simulink model "pid_teta_x"  (R2017b)
settings: Solver=VariableStepAuto  StartTime=0.0  StopTime=3  RelTol=1e-3
libraries: simulink_extras x4, simulink x2
settings Model: Creator=Iman  LastModifiedBy=Iman

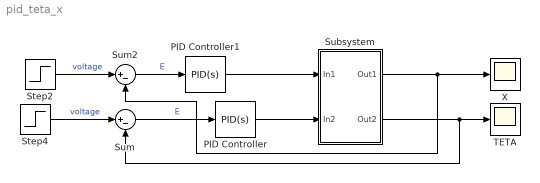
== system pid_teta_x ==
  PID Controller : simulink/Continuous/PID Controller  Controller=PID  TimeDomain=Continuous-time  SampleTime=-1  IntegratorMethod=Forward Euler  FilterMethod=Forward Euler  Form=Parallel  UseFilter=on  ControllerParametersSource=internal  P=-5528615749.16479  I=-14443726305.4223  D=1766735.00522136  N=3129.2840934411  InitialConditionSource=internal  InitialConditionForIntegrator=0  InitialConditionForFilter=0  ExternalReset=none  LimitOutput=off  UpperSaturationLimit=inf  LowerSaturationLimit=-inf  LinearizeAsGain=on  AntiWindupMode=none  Kb=1  TrackingMode=off  Kt=1  PParamMin=[]  PParamMax=[]  IParamMin=[]  IParamMax=[]  DParamMin=[]  DParamMax=[]  NParamMin=[]  NParamMax=[]  KbParamMin=[]  KbParamMax=[]  KtParamMin=[]  KtParamMax=[]  POutMin=[]  POutMax=[]  IOutMin=[]  IOutMax=[]  DOutMin=[]  DOutMax=[]  NOutMin=[]  NOutMax=[]  KbOutMin=[]  KbOutMax=[]  KtOutMin=[]  KtOutMax=[]  IntegratorOutMin=[]  IntegratorOutMax=[]  FilterOutMin=[]  FilterOutMax=[]  SumOutMin=[]  SumOutMax=[]  SumI1OutMin=[]  SumI1OutMax=[]  SumI2OutMin=[]  SumI2OutMax=[]  SumI3OutMin=[]  SumI3OutMax=[]  SumDOutMin=[]  SumDOutMax=[]  SaturationOutMin=[]  SaturationOutMax=[]  IntegratorContinuousStateAttributes=''  IntegratorStateMustResolveToSignalObject=off  IntegratorRTWStateStorageClass=Auto  FilterContinuousStateAttributes=''  FilterStateMustResolveToSignalObject=off  FilterRTWStateStorageClass=Auto  DifferentiatorICPrevScaledInput=0  DifferentiatorOutMin=[]  DifferentiatorOutMax=[]  InitialConditionSetting=State (most efficient)  FilterDiffOutCoefMin=[]  FilterDiffOutCoefMax=[]  SumDenOutMin=[]  SumDenOutMax=[]  SumNumOutMin=[]  SumNumOutMax=[]  ReciprocalOutMin=[]  ReciprocalOutMax=[]  DivideOutMin=[]  DivideOutMax=[]  TunerSelectOption=Transfer Function Based (PID Tuner App)
  PID Controller1 : simulink/Continuous/PID Controller  Controller=PID  TimeDomain=Continuous-time  SampleTime=-1  IntegratorMethod=Forward Euler  FilterMethod=Forward Euler  Form=Parallel  UseFilter=on  ControllerParametersSource=internal  P=85.1454280076779  I=92.389206029507  D=18.0340374207708  N=3627.1106134896  InitialConditionSource=internal  InitialConditionForIntegrator=0  InitialConditionForFilter=0  ExternalReset=none  LimitOutput=off  UpperSaturationLimit=inf  LowerSaturationLimit=-inf  LinearizeAsGain=on  AntiWindupMode=none  Kb=1  TrackingMode=off  Kt=1  PParamMin=[]  PParamMax=[]  IParamMin=[]  IParamMax=[]  DParamMin=[]  DParamMax=[]  NParamMin=[]  NParamMax=[]  KbParamMin=[]  KbParamMax=[]  KtParamMin=[]  KtParamMax=[]  POutMin=[]  POutMax=[]  IOutMin=[]  IOutMax=[]  DOutMin=[]  DOutMax=[]  NOutMin=[]  NOutMax=[]  KbOutMin=[]  KbOutMax=[]  KtOutMin=[]  KtOutMax=[]  IntegratorOutMin=[]  IntegratorOutMax=[]  FilterOutMin=[]  FilterOutMax=[]  SumOutMin=[]  SumOutMax=[]  SumI1OutMin=[]  SumI1OutMax=[]  SumI2OutMin=[]  SumI2OutMax=[]  SumI3OutMin=[]  SumI3OutMax=[]  SumDOutMin=[]  SumDOutMax=[]  SaturationOutMin=[]  SaturationOutMax=[]  IntegratorContinuousStateAttributes=''  IntegratorStateMustResolveToSignalObject=off  IntegratorRTWStateStorageClass=Auto  FilterContinuousStateAttributes=''  FilterStateMustResolveToSignalObject=off  FilterRTWStateStorageClass=Auto  DifferentiatorICPrevScaledInput=0  DifferentiatorOutMin=[]  DifferentiatorOutMax=[]  InitialConditionSetting=State (most efficient)  FilterDiffOutCoefMin=[]  FilterDiffOutCoefMax=[]  SumDenOutMin=[]  SumDenOutMax=[]  SumNumOutMin=[]  SumNumOutMax=[]  ReciprocalOutMin=[]  ReciprocalOutMax=[]  DivideOutMin=[]  DivideOutMax=[]  TunerSelectOption=Transfer Function Based (PID Tuner App)
  Step2 : Step  Time=0  SampleTime=0.1
  Step4 : Step  Time=0  SampleTime=0.1
  Subsystem : Subsystem
  Sum : Sum  Inputs=|+-
  Sum2 : Sum  Inputs=|+-
  TETA : Scope
  X : Scope
  wires:
  Step4/1 -> Sum/1  "voltage"
  Sum/1 -> PID Controller/1  "E"
  Subsystem/1(Out1) -> Sum2/2, X/1
  Subsystem/2(Out2) -> TETA/1, Sum/2
  PID Controller/1 -> Subsystem/2(In2)
  PID Controller1/1 -> Subsystem/1(In1)
  Step2/1 -> Sum2/1  "voltage"
  Sum2/1 -> PID Controller1/1  "E"

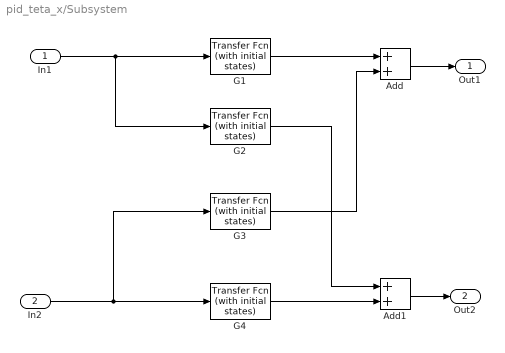
== system pid_teta_x/Subsystem ==
  In1 : Inport
  In2 : Inport  Port=2
  Add : Sum
  Add1 : Sum
  G1 : simulink_extras/Additional Linear/Transfer Fcn (with initial states)  N="[1275  2.924e06  1.801e11  3.448e14  -1.264e16 -2.579e16  -5.022e04].*(-1)"  D="[1  5372   2.732e08  1.366e12  1.934e16  8.664e19  1.019e23  -7.863e21 5.559e24 0 ]"  X0=0
  G2 : simulink_extras/Additional Linear/Transfer Fcn (with initial states)  N="[-1.932e04   4.666e07  2.734e12  5.557e15  4.591e17  2.648e06].*(-1)"  D="[1  5372   2.732e08  1.366e12  1.934e16  8.664e19  1.019e23  -7.863e21 5.559e24 0 ]"  X0=0
  G3 : simulink_extras/Additional Linear/Transfer Fcn (with initial states)  N="[1275  2.924e06  1.801e11  3.448e14  -1.264e16 -2.579e16  -5.022e04].*(-1)"  D="[1  5372   2.732e08  1.366e12  1.934e16  8.664e19  1.019e23  -7.863e21 5.559e24 0 ]"  X0=0
  G4 : simulink_extras/Additional Linear/Transfer Fcn (with initial states)  N="[-1.932e04   4.666e07  2.734e12  5.557e15  4.591e17  2.648e06].*(-1)"  D="[1  5372   2.732e08  1.366e12  1.934e16  8.664e19  1.019e23  -7.863e21 5.559e24 0 ]"  X0=0
  Out1 : Outport
  Out2 : Outport  Port=2
  wires:
  Add1/1 -> Out2/1
  Add/1 -> Out1/1
  G1/1 -> Add/1
  In1/1 -> G2/1, G1/1
  In2/1 -> G4/1, G3/1
  G3/1 -> Add/2
  G2/1 -> Add1/1
  G4/1 -> Add1/2
